simulink model "Lab_Mechanical_System"  (R2018a)
settings: Solver=VariableStepAuto  StartTime=0.0  StopTime=200  RelTol=1e-3
libraries: dspsrcs4 x1
settings Model: Creator=samak-twins  LastModifiedBy=samak

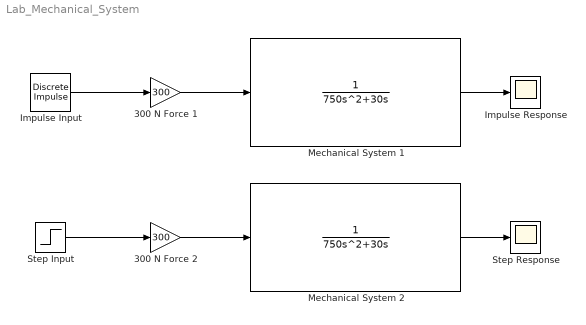
== system Lab_Mechanical_System ==
  300 N Force 1 : Gain  Gain=300
  300 N Force 2 : Gain  Gain=300
  Impulse Input : dspsrcs4/Discrete  Impulse  Delay=0  SampleTime=1  FrameSample=1  OutputFrames=off  dataType=double  isSigned=on  wordLen=16  udDataType=sfix(16)  fracBitsMode=Best precision  numFracBits=15  OutDataTypeStr=double  LastOutDataTypeStr=double
  Impulse Response : Scope
  Mechanical System 1 : TransferFcn  Denominator=[750 30 0]
  Mechanical System 2 : TransferFcn  Denominator=[750 30 0]
  Step Input : Step  Time=0  SampleTime=0
  Step Response : Scope
  wires:
  Mechanical System 1/1 -> Impulse Response/1
  Mechanical System 2/1 -> Step Response/1
  Impulse Input/1 -> 300 N Force 1/1
  300 N Force 1/1 -> Mechanical System 1/1
  Step Input/1 -> 300 N Force 2/1
  300 N Force 2/1 -> Mechanical System 2/1
